simulink model "adrc_matlab_model"  (R2019b)
settings: Solver=FixedStepDiscrete  StartTime=0.0  StopTime=5  FixedStep=Ts  RelTol=1e-3
PreLoadFcn:
  | Ts = 0.001;
  | Inertia = 2;
InitFcn:
  | Ts = 0.001;
  | Inertia = 2;
undefined symbols (not defined in the file): DiscIntNeverNeededParam
libraries: adrc x6, motion x1
settings Model: Creator=Kamran  LastModifiedBy=Kamran
settings SimscapeCC: SimscapeNormalizeSystem=off

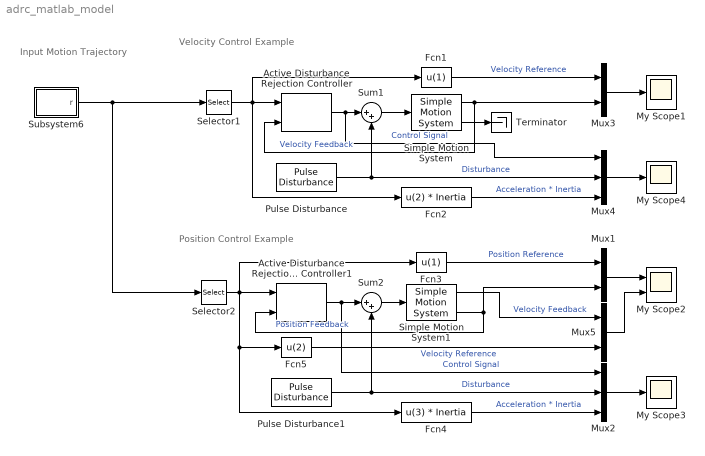
== system adrc_matlab_model ==
  note: Input Motion
      | Trajectory
  note: Position Control Example
  note: Velocity Control Example
  Active Disturbance Rejection Controller : adrc/Active Disturbance Rejection Controller  b=1/Inertia  w=40  n=1  sat=3
  Active Disturbance Rejection Controller1 : adrc/Active Disturbance Rejection Controller  b=1/Inertia  w=40  n=2  sat=3
  Fcn1 : Fcn  Expr=u(1)
  Fcn2 : Fcn  Expr=u(2) * Inertia
  Fcn3 : Fcn  Expr=u(1)
  Fcn4 : Fcn  Expr=u(3) * Inertia
  Fcn5 : Fcn  Expr=u(2)
  Mux1 : Mux  Inputs=2
  Mux2 : Mux  Inputs=3
  Mux3 : Mux  Inputs=2
  Mux4 : Mux  Inputs=3
  Mux5 : Mux  Inputs=2
  My Scope1 : Scope
  My Scope2 : Scope  NumInputPorts=2
  My Scope3 : Scope
  My Scope4 : Scope
  Pulse Disturbance : adrc/Pulse Disturbance  d=2.5  t=0.05  w=2  e=on
  Pulse Disturbance1 : adrc/Pulse Disturbance  d=2.5  t=0.05  w=2  e=on
  Selector1 : Selector  InputPortWidth=3  IndexOptions=Index vector (dialog)  Indices=[2 3]  OutputSizes=1
  Selector2 : Selector  InputPortWidth=3  IndexOptions=Index vector (dialog)  Indices=[1 2 3]  OutputSizes=1
  Simple Motion System : adrc/Simple Motion System  I=Inertia  K=0.2  Taw=1e-3  Ts=Ts
  Simple Motion System1 : adrc/Simple Motion System  I=Inertia  K=0.2  Taw=1e-3  Ts=Ts
  Subsystem6 : Subsystem
      mask Display: disp("Profile")
  Sum1 : Sum  Inputs=|++
  Sum2 : Sum  Inputs=|++
  Terminator : Terminator
  wires:
  Sum1/1 -> Simple Motion System/1
  Simple Motion System/1 -> Mux3/2, Active Disturbance Rejection Controller/2  "Velocity Feedback"
  Fcn1/1 -> Mux3/1  "Velocity Reference"
  Active Disturbance Rejection Controller/1 -> Sum1/1, Mux4/1  "Control Signal"
  Selector1/1 -> Active Disturbance Rejection Controller/1, Fcn2/1, Fcn1/1
  Mux4/1 -> My Scope4/1
  Mux3/1 -> My Scope1/1
  Fcn2/1 -> Mux4/3  "Acceleration * Inertia"
  Pulse Disturbance/1 -> Mux4/2, Sum1/2  "Disturbance"
  Simple Motion System1/2 -> Active Disturbance Rejection Controller1/2, Mux1/2  "Position Feedback"
  Sum2/1 -> Simple Motion System1/1
  Simple Motion System1/1 -> Mux5/1  "Velocity Feedback"
  Active Disturbance Rejection Controller1/1 -> Mux2/1, Sum2/1  "Control Signal"
  Mux2/1 -> My Scope3/1
  Mux5/1 -> My Scope2/2
  Fcn5/1 -> Mux5/2  "Velocity Reference"
  Fcn4/1 -> Mux2/3  "Acceleration * Inertia"
  Fcn3/1 -> Mux1/1  "Position Reference"
  Selector2/1 -> Fcn4/1, Fcn5/1, Active Disturbance Rejection Controller1/1, Fcn3/1
  Pulse Disturbance1/1 -> Sum2/2, Mux2/2  "Disturbance"
  Mux1/1 -> My Scope2/1
  Subsystem6/1(r) -> Selector2/1, Selector1/1
  Simple Motion System/2 -> Terminator/1

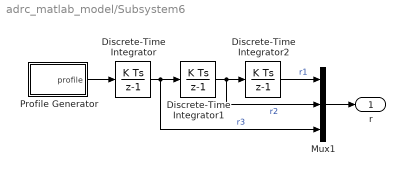
== system adrc_matlab_model/Subsystem6 ==
  Discrete-Time Integrator : DiscreteIntegrator  SampleTime=-1  ICPrevOutput=DiscIntNeverNeededParam  ICPrevScaledInput=DiscIntNeverNeededParam
  Discrete-Time Integrator1 : DiscreteIntegrator  SampleTime=-1  ICPrevOutput=DiscIntNeverNeededParam  ICPrevScaledInput=DiscIntNeverNeededParam
  Discrete-Time Integrator2 : DiscreteIntegrator  SampleTime=-1  ICPrevOutput=DiscIntNeverNeededParam  ICPrevScaledInput=DiscIntNeverNeededParam
  Mux1 : Mux  Inputs=3
  Profile Generator : Subsystem  BlockChoice=Jerk
      link override Jerk: t0=1  x=2  a=2  j=3  Ts=Ts
      settings: AttributesFormatString=%<BlockChoice>  TemplateBlock=motion/Profile Generators/Profile Generator  MemberBlocks=Acceleration,Derivative of Jerk,Jerk,dJerk with error correction
  r : Outport
  wires:
  Profile Generator/1(profile) -> Discrete-Time Integrator/1
  Discrete-Time Integrator1/1 -> Mux1/2, Discrete-Time Integrator2/1  "r2"
  Discrete-Time Integrator/1 -> Mux1/3, Discrete-Time Integrator1/1  "r3"
  Mux1/1 -> r/1
  Discrete-Time Integrator2/1 -> Mux1/1  "r1"

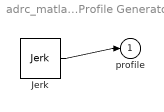
== system adrc_matlab_model/Subsystem6/Profile Generator ==
  Jerk : motion/Profile Generators/Jerk  t0=1  x=2  v=1  a=2  j=3  Ts=Ts
  profile : Outport
  wires:
  Jerk/1 -> profile/1
